simulink library "csc_cmp_command_mode_process_lib"  (R2014b)
settings: Solver=ode45  StartTime=0.0  StopTime=10.0  RelTol=1e-3
values from neighbouring files (symbols this model uses):
  csc_cmp_dt = fsw_dt    [csc_cmp_command_mode_process_init.m]
libraries: util_info_lib x1, csu_cml_command_latch_lib x1
settings Model: Creator=mstewart  LastModifiedBy=mstewart

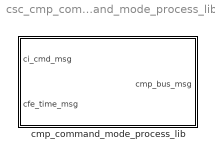
== system csc_cmp_command_mode_process_lib ==
  cmp_command_mode_process_lib : Subsystem  Tag=OFSW  TreatAsAtomicUnit=on  SystemSampleTime=csc_cmp_dt

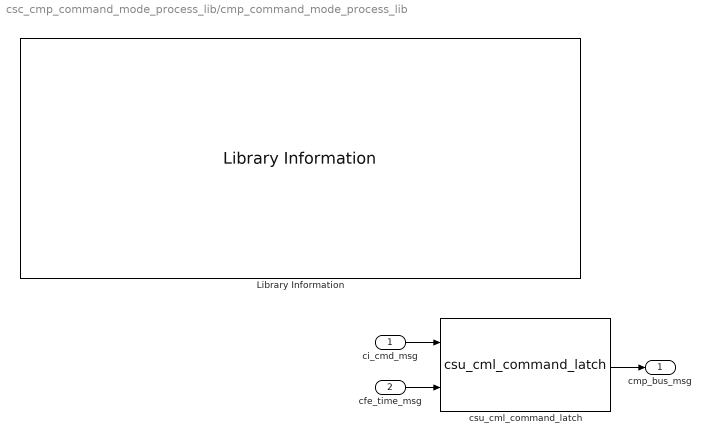
== system csc_cmp_command_mode_process_lib/cmp_command_mode_process_lib ==
  ci_cmd_msg : Inport  OutDataTypeStr=Bus: ci_cmd_msg
  cfe_time_msg : Inport  Port=2  OutDataTypeStr=Bus: cfe_time_msg
  Library Information : util_info_lib/Library Information  owner='NONE'
  csu_cml_command_latch : csu_cml_command_latch_lib/csu_cml_command_latch
  cmp_bus_msg : Outport  OutDataTypeStr=Bus: cmp_bus_msg
  wires:
  csu_cml_command_latch/1 -> cmp_bus_msg/1
  ci_cmd_msg/1 -> csu_cml_command_latch/1
  cfe_time_msg/1 -> csu_cml_command_latch/2
